simulink model "rocketprojSimulink"  (R2025a)
settings: Solver=ode1  StartTime=0.0  StopTime=60  FixedStep=.02  MaxStep=.01  RelTol=1e-3
values from neighbouring files (symbols this model uses):
  a = .0045    (= 0.0045)    [newRocketProj.m]
  g = 9.81    [newRocketProj.m]
  mProp = 0.5    [newRocketProj.m]
  mTotal = mDry + mProp    (= 1.55)    [newRocketProj.m]
libraries: simulink x1, aerolibatmos2 x1, dspadpt3 x1
settings Model: Creator=ferrer3  LastModifiedBy=ferrer3

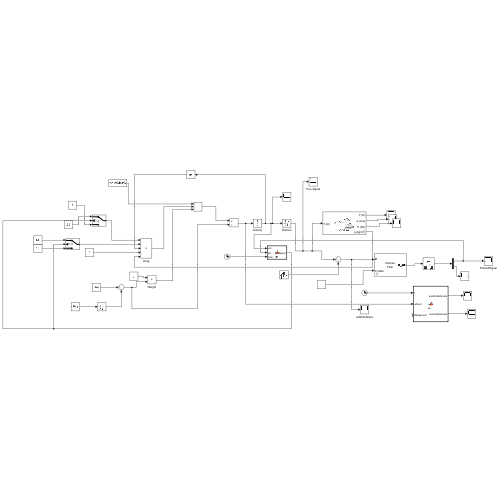
[thumbnail: Simulink's stored preview of the top-level diagram]
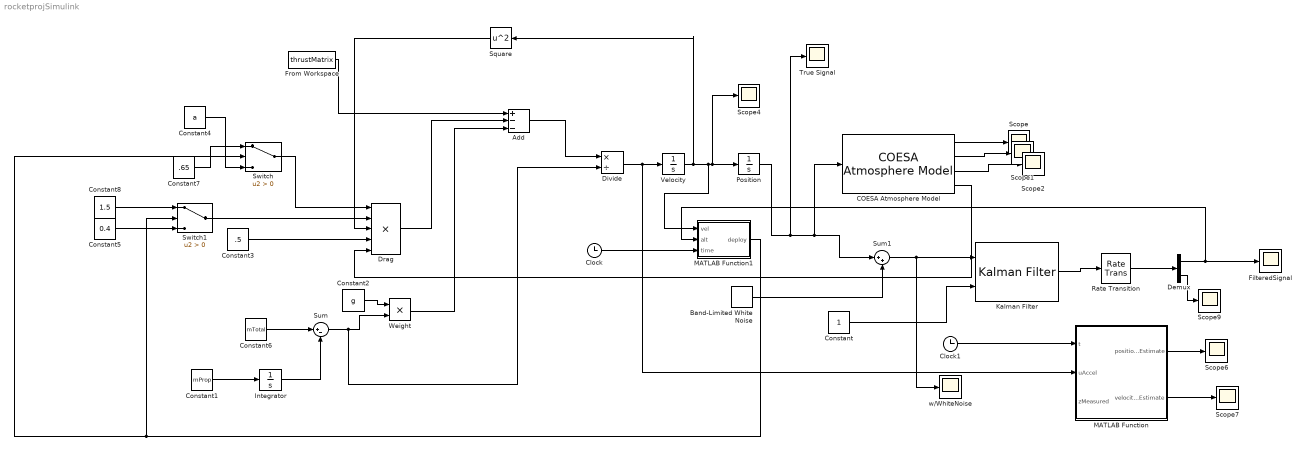
== system rocketprojSimulink ==
  Add : Sum  Inputs=+--
  Band-Limited White Noise : simulink/Sources/Band-Limited White Noise  Cov=[0.1]  Ts=0.1  seed=[23341]
  COESA Atmosphere Model : aerolibatmos2/COESA Atmosphere Model  units=Metric (MKS)  spec=1976 COESA-extended U.S. Standard Atmosphere  model=Profile  profile_var=High temperature  profile_percent=1%  profile_alt=5 km (16404 ft)  envelope_var=High temperature  envelope_percent=1%  action=Warning
  Clock : Clock
  Clock1 : Clock
  Constant : Constant
  Constant1 : Constant  Value=mProp
  Constant2 : Constant  Value=g
  Constant3 : Constant  Value=.5
  Constant4 : Constant  Value=a
  Constant5 : Constant  Value=0.4
  Constant6 : Constant  Value=mTotal
  Constant7 : Constant  Value=.65
  Constant8 : Constant  Value=1.5
  Demux : Demux  Outputs=2
  Divide : Product  Inputs=*/
  Drag : Product  Inputs=5
  FilteredSignal : Scope
      settings: ActiveDisplayYMinimum=378.34853343025895  ActiveDisplayYMaximum=392.26424049056072  DataLoggingVariableName=ScopeData8
  From Workspace : FromWorkspace  VariableName=thrustMatrix  OutputAfterFinalValue=Setting to zero
  Integrator : Integrator  LimitOutput=on  LowerSaturationLimit=0
  Kalman Filter : dspadpt3/Kalman Filter  num_targets=1  sourceEnable=Specify via input port <Enable>  isReset=on  X=[0; 0]  P=eye(2)  A=[1, 0.02; 0,1]  sourceMeasure=Specify via dialog  H=[1,0]  Q=diag([0.01,0.1])  R=[5.0]  isOutputEstMeasure=off  isOutputEstState=on  isOutputEstError=off  isOutputPrdMeasure=off  isOutputPrdState=off  isOutputPrdError=off
  MATLAB Function : MATLAB Function  TreatAsAtomicUnit=on  SystemSampleTime=.01
  MATLAB Function1 : MATLAB Function  TreatAsAtomicUnit=on  SystemSampleTime=.01
  Position : Integrator  LimitOutput=on  UpperSaturationLimit=1000000000000  LowerSaturationLimit=0
  Rate Transition : RateTransition  OutPortSampleTime=.01
  Scope{,1..2,4,6..7,9} (7 alike) : Scope
      Scope settings: ActiveDisplayYMinimum=-1  ActiveDisplayYMaximum=1
      Scope2 settings: ActiveDisplayYMinimum=-1  ActiveDisplayYMaximum=1  DataLoggingVariableName=ScopeData2
      Scope4 settings: ActiveDisplayYMinimum=-193.36455635279947  ActiveDisplayYMaximum=113.06270413093722  DataLoggingVariableName=ScopeData4
      Scope6 settings: ActiveDisplayYMinimum=-8.2331618125127716E+10  ActiveDisplayYMaximum=1.6586992976218086E+10  DataLoggingVariableName=ScopeData5
      Scope7 settings: ActiveDisplayYMinimum=-1.1865935759258087E+11  ActiveDisplayYMaximum=1.3891206700803316E+10  DataLoggingVariableName=ScopeData6
      Scope9 settings: ActiveDisplayYMinimum=-26.538982038045582  ActiveDisplayYMaximum=71.561651306120268  DataLoggingVariableName=ScopeData9
  Square : Math  Operator=square
  Sum : Sum  Inputs=|+-
  Sum1 : Sum  Inputs=|++
  Switch : Switch  Criteria=u2 > Threshold  SaturateOnIntegerOverflow=off  InputSameDT=off
  Switch1 : Switch  Criteria=u2 > Threshold  SaturateOnIntegerOverflow=off  InputSameDT=off
  True Signal : Scope
      settings: ActiveDisplayYMinimum=-950.72630250397822  ActiveDisplayYMaximum=729.8927526854626  DataLoggingVariableName=ScopeData3
  Velocity : Integrator
  Weight : Product
  w/WhiteNoise : Scope
      settings: ActiveDisplayYMinimum=-81.3747416993083  ActiveDisplayYMaximum=708.93923386036909  DataLoggingVariableName=ScopeData7
  wires:
  Add/1 -> Divide/1
  Constant2/1 -> Weight/1
  Sum/1 -> Divide/2, Weight/2
  Weight/1 -> Add/3
  Divide/1 -> MATLAB Function/2(uAccel), Velocity/1
  Drag/1 -> Add/2
  COESA Atmosphere Model/4 -> Drag/5
  Velocity/1 -> Square/1, MATLAB Function1/1(vel), Position/1, Scope4/1
  Constant3/1 -> Drag/4
  Square/1 -> Drag/3
  From Workspace/1 -> Add/1
  COESA Atmosphere Model/1 -> Scope/1
  COESA Atmosphere Model/2 -> Scope1/1
  COESA Atmosphere Model/3 -> Scope2/1
  Position/1 -> True Signal/1, COESA Atmosphere Model/1, Sum1/1
  Constant1/1 -> Integrator/1
  Integrator/1 -> Sum/2
  Constant6/1 -> Sum/1
  Band-Limited White Noise/1 -> Sum1/2
  Sum1/1 -> w/WhiteNoise/1, Kalman Filter/1
  MATLAB Function/1(positionEstimate) -> Scope6/1
  MATLAB Function/2(velocityEstimate) -> Scope7/1
  Constant/1 -> Kalman Filter/2
  Demux/1 -> MATLAB Function1/2(alt), FilteredSignal/1
  Demux/2 -> Scope9/1
  Rate Transition/1 -> Demux/1
  Kalman Filter/1 -> Rate Transition/1
  Clock/1 -> MATLAB Function1/3(time)
  MATLAB Function1/1(deploy) -> Switch/2, Switch1/2
  Switch/1 -> Drag/1
  Constant4/1 -> Switch/3
  Constant7/1 -> Switch/1
  Switch1/1 -> Drag/2
  Constant5/1 -> Switch1/3
  Constant8/1 -> Switch1/1
  Clock1/1 -> MATLAB Function/1(t)

== matlab function rocketprojSimulink/MATLAB Function1 ==
  data: vel input; deploy output; alt input; time input
function deploy = fcn(vel, alt, time)
persistent isDeployed;

if isempty(isDeployed)
    isDeployed = 0;
end

if time > 10 && alt > 5 && vel <= 0
    isDeployed = 1;
end 

deploy = isDeployed;
end

== matlab function rocketprojSimulink/MATLAB Function ==
  data: t input; uAccel input; zMeasured input; positionEstimate output; velocityEstimate output
function [positionEstimate, velocityEstimate] = fcn(t, uAccel,zMeasured)
% These values stay the same across all of the time steps of the simulation
persistent xHat errorCovar
% xHat is the state estimate, or the best guess as to where we are
% errorCovar is the uncertainty of the current state estimate (xHat)
% High value means it is very uncertain and a low value means confident

% Tuning parameters( Higher value means more uncertainty )
% (Q) Looks for external forces, unpredictable things, and the model itself
persistent systemCovar
% (R) Sees how unreliable the sensor readings are
persistent measureCovar


persistent lastTimeUpdate
persistent initialized



% BTW covariance measures how much variables change together

% Initialization when xHat doesn't have a value (i.e. start of sim)
if isempty(initialized)
    % Initializes it as 0 position and 0 velocity
    xHat = [0; 0];
    % eye command creates an identity matrix, the number means num x num
    % in this case it creates a 2x2 identity matrix 
    errorCovar = eye(2);
    % initializing model confidence covariance for the system 
    % Is a matrix because we have different covariant values for pos & vel
    systemCovar = diag([0.01, 0.1]);
    % initializing sensor confidence covariance for the system
    % JUST KNOW: if we are using multiple sensors, then we would use a 
    % matrix, but in this case we are only using altitude sensor, so
    % it can just stay as a single number
    measureCovar = 5.0;
    % timeStep, we set this to .01 in this case
    lastTimeUpdate = 0;
    initialized = true;
end

sensorSampleTime = .02;
if (t - lastTimeUpdate) >= sensorSampleTime
    dt = t - lastTimeUpdate;
    lastTimeUpdate = t;

    % Step 1: Predict the step

    % State transition matrix, every time we take a step (dt), we use this to 
    % calculate where we are next, we leave the acceleration to B (control
    % input matrix)
    % newPosition  = oldPosition + (velocity * dt)
    A = [1, dt;
         0, 1 ];
    
    % Control input matrix, tells the program how acceleration affects the pos
    % and vel over dt
    % x_k+1 = Ax_k + Bu_k
    B = [0.5 * dt^2;
        dt];
    % Make a prediction as to where the x should be
    xPrediction = A * xHat + B * uAccel;
    
    % Make a prediction on the error covariance 
    errorPrediction = A * errorCovar * A' + systemCovar;
    
    % Step 2: Update and correct the step
    % Measurement Matrix: This gives us the position from the sensor
    C = [1,0];
    
    % yTilde is the residual. It is the difference between the actual
    % measurement and the expected measurement
    yTilde = zMeasured - (C * xPrediction);
    
    % Innovation covariance is the total uncertainty of the residual
    S = C * errorPrediction * C' + measureCovar;
    
    % Kalman gain: Figures out how much weight should be given to the new
    % measurement vs the prediction 
    K = errorPrediction * C' / S;
    
    % Update our state estimate with the measurement 
    xHat = xPrediction + K * yTilde;
    
    % Update our error covariance 
    errorCovar = (eye(2) - K * C) * errorPrediction;
end



positionEstimate = xHat(1);
velocityEstimate = xHat(2);
end
